simulink model "desacoplador"  (R2017a)
settings: Solver=VariableStepAuto  StartTime=0.0  StopTime=10.0  RelTol=1e-3
settings Model: Creator=Lizeth P. Guzman  LastModifiedBy=Lizeth P. Guzman

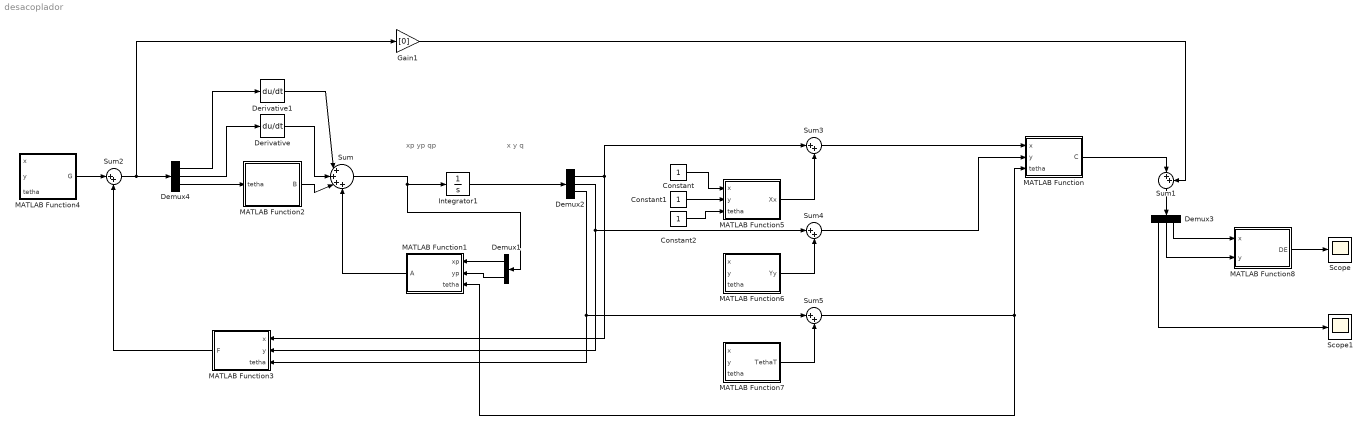
== system desacoplador ==
  note: x
      | y
      | q
  note: xp
      | yp
      | qp
  Constant : Constant
  Constant1 : Constant
  Constant2 : Constant
  Demux1 : Demux  Outputs=2
  Demux2 : Demux  Outputs=3
  Demux3 : Demux  Outputs=3
  Demux4 : Demux  Outputs=3
  Derivative : Derivative
  Derivative1 : Derivative
  Gain1 : Gain  Gain=[0]
  Integrator1 : Integrator
  MATLAB Function : MATLAB Function  TreatAsAtomicUnit=on
  MATLAB Function1 : MATLAB Function  TreatAsAtomicUnit=on
  MATLAB Function2 : MATLAB Function  TreatAsAtomicUnit=on
  MATLAB Function3 : MATLAB Function  TreatAsAtomicUnit=on
  MATLAB Function4 : MATLAB Function  TreatAsAtomicUnit=on
  MATLAB Function5 : MATLAB Function  TreatAsAtomicUnit=on
  MATLAB Function6 : MATLAB Function  TreatAsAtomicUnit=on
  MATLAB Function7 : MATLAB Function  TreatAsAtomicUnit=on
  MATLAB Function8 : MATLAB Function  TreatAsAtomicUnit=on
  Scope : Scope
  Scope1 : Scope
  Sum : Sum  Inputs=|++++
  Sum{1..5} (5 alike) : Sum  Inputs=|++
  wires:
  Sum/1 -> Integrator1/1, Demux1/1
  MATLAB Function4/1(G) -> Sum2/1
  MATLAB Function/1(C) -> Sum1/1
  Gain1/1 -> Sum1/2
  Sum5/1 -> MATLAB Function/3(tetha), MATLAB Function1/3(tetha)
  Integrator1/1 -> Demux2/1
  Demux1/2 -> MATLAB Function1/2(yp)
  Demux1/1 -> MATLAB Function1/1(xp)
  Sum2/1 -> Gain1/1, Demux4/1
  MATLAB Function3/1(F) -> Sum2/2
  Sum1/1 -> Demux3/1
  Demux3/1 -> Scope1/1
  Demux3/3 -> MATLAB Function8/1(x)
  Demux3/2 -> MATLAB Function8/2(y)
  Demux2/2 -> MATLAB Function3/2(y), Sum4/1
  MATLAB Function5/1(Xx) -> Sum3/2
  Demux2/1 -> MATLAB Function3/1(x), Sum3/1
  MATLAB Function7/1(TethaT) -> Sum5/2
  MATLAB Function6/1(Yy) -> Sum4/2
  Demux2/3 -> Sum5/1, MATLAB Function3/3(tetha)
  Sum3/1 -> MATLAB Function/1(x)
  Sum4/1 -> MATLAB Function/2(y)
  MATLAB Function8/1(DE) -> Scope/1
  Constant/1 -> MATLAB Function5/1(x)
  Constant1/1 -> MATLAB Function5/2(y)
  Constant2/1 -> MATLAB Function5/3(tetha)
  Demux4/3 -> MATLAB Function2/1(tetha)
  MATLAB Function1/1(A) -> Sum/4
  MATLAB Function2/1(B) -> Sum/3
  Demux4/1 -> Derivative1/1
  Demux4/2 -> Derivative/1
  Derivative/1 -> Sum/2
  Derivative1/1 -> Sum/1

== matlab function desacoplador/MATLAB Function1 ==
  data: xp input; A output; yp input; tetha input
function A = fcn(xp, yp, tetha)
%#codegen
v=sqrt((xp^2)+(yp^2));
w=atan2(yp,xp);
d=1;


A=[0 0 -v*sin(tetha)-(d*w*cos(tetha));
   0 0  v*cos(tetha)-(d*w*sin(tetha));
   0 0  0 ];

== matlab function desacoplador/MATLAB Function ==
  data: x input; C output; y input; tetha input
function C = fcn(x, y, tetha)
%#codegen

C=[(x)/(((x^2)+(y^2))^(1/2)) (y)/(((x^2)+(y^2))^(1/2)) 0;
    0 0 1 ];

== matlab function desacoplador/MATLAB Function2 ==
  data: B output; tetha input
function B = fcn(tetha)
%#codegen
d=1;
B=[cos(tetha) -d*sin(tetha);
   sin(tetha)  d*cos(tetha);
   0           1];

== matlab function desacoplador/MATLAB Function3 ==
  data: x input; F output; y input; tetha input
function F = fcn(x, y, tetha)
%#codegen
v=sqrt((x^2)+(y^2));
w=atan2(y,x);
d=1;
 
F=[ 0, 0, -((x^2 + y^2)^(1/2)*((x*(v*sin(tetha) + d*w*cos(tetha)))/(x^2 + y^2)^(1/2) - (y*(v*cos(tetha) - d*w*sin(tetha)))/(x^2 + y^2)^(1/2)))/(x*cos(tetha) + y*sin(tetha));
    0, 0,                                                                                                                                                                  0];

== matlab function desacoplador/MATLAB Function4 ==
  data: x input; y input; G output; tetha input
function  G = fcn(x, y, tetha)
%#codegen
d=1;
G =[ (x^2 + y^2)^(1/2)/(x*cos(tetha) + y*sin(tetha)), -(d*(y*cos(tetha) - x*sin(tetha)))/(x*cos(tetha) + y*sin(tetha));
                                                0,                                                                1];

== matlab function desacoplador/MATLAB Function5 ==
  data: x input; Xx output; y input; tetha input
function Xx = fcn(x, y, tetha)
%#codegen

== matlab function desacoplador/MATLAB Function6 ==
  data: x input; Yy output; y input; tetha input
function Yy = fcn(x, y, tetha)
%#codegen

== matlab function desacoplador/MATLAB Function7 ==
  data: x input; TethaT output; y input; tetha input
function TethaT = fcn(x, y, tetha)
%#codegen

== matlab function desacoplador/MATLAB Function8 ==
  data: x input; DE output; y input
function DE = fcn(x, y)
%#codegen

DE=sqrt((x^2)+(y^2));
